simulink model "CANTXcommunicationunit_2"  (R2024a)
settings: Solver=VariableStepAuto  StartTime=0.0  StopTime=10.0  RelTol=1e-3
undefined symbols (not defined in the file or in its folder): canChannel
libraries: canlib x2, canmsglib x1
settings Model: DataDictionary=BMS_System_dict1.sldd  Creator=hirah  LastModifiedBy=hirah

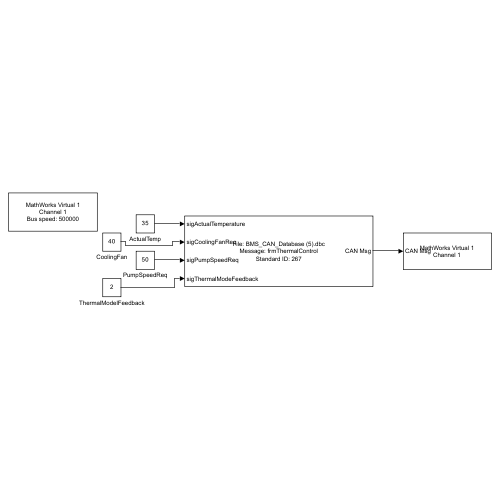
[thumbnail: Simulink's stored preview of the top-level diagram]
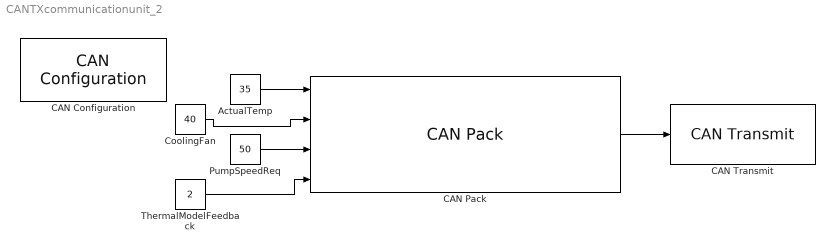
== system CANTXcommunicationunit_2 ==
  ActualTemp : Constant  Value=35  OutDataTypeStr=uint8
  CAN Configuration : canlib/CAN Configuration  BlockHandle=657.0001  Device=MathWorks Virtual 1 (Channel 1)  DeviceMenu=MathWorks Virtual 1 (Channel 1)  ObjConstructor=canChannel('MathWorks', 'Virtual 1', 1)  BusSpeed=500000  EnableBitParameters=off  AckMode=Normal
  CAN Pack : canmsglib/CAN Pack  CANdbFile=C:\Users\hirah\Downloads\BMS_CAN_Database (5).dbc  MsgList=frmThermalControl  MsgName=frmThermalControl  MsgIDType=Standard (11-bit identifier)  MsgIdentifier=267  MsgLength=4  Remote=off  ApplyMinMax=off  BusOutput=off  SignalInfo={'sigActualTemperature','24','8','LE','unsigned','Standard','0','1','0','0','100';'sigCoolingFanReq','0','8','LE','unsigned','Standard','0','1','0','0','100';'sigPumpSpeedReq','8','8','LE','unsigned','Standard','0','1','0','0','100';'sigThermalModeFeedback','16','8','LE','unsigned','Standard','0','1','0','0','4'}
      settings: LibrarySourceBlock=canlib/CAN Pack  DataFormat=CANdb specified signals
  CAN Transmit : canlib/CAN Transmit  BlockHandle=664.0001  Device=MathWorks Virtual 1 (Channel 1)  DeviceMenu=MathWorks Virtual 1 (Channel 1)  ObjConstructor=canChannel('MathWorks', 'Virtual 1', 1)  EnableEventTransmit=off  EnablePeriodicTransmit=off  MessagePeriod=1.000
  CoolingFan : Constant  Value=40  OutDataTypeStr=uint8
  PumpSpeedReq : Constant  Value=50  OutDataTypeStr=uint8
  ThermalModelFeedback : Constant  Value=2  OutDataTypeStr=uint8
  wires:
  CAN Pack/1 -> CAN Transmit/1
  ActualTemp/1 -> CAN Pack/1
  CoolingFan/1 -> CAN Pack/2
  PumpSpeedReq/1 -> CAN Pack/3
  ThermalModelFeedback/1 -> CAN Pack/4
